simulink model "BuildYourOwnMSD"  (R2024a)
settings: Solver=VariableStepAuto  StartTime=0.0  StopTime=50  MaxStep=0.1  RelTol=1e-3
PreLoadFcn:
  | load Data\MSDParams.mat
undefined symbols (not defined in the file): A, Cd, g, L, m, rho, xdot
libraries: fl_lib x8, nesl_utility x4
CloseFcn:
  | clear
settings Model: Creator=callie  LastModifiedBy=vboutrou
settings DataIOCC: ReturnWorkspaceOutputsName=out3
settings ConfigComp: CovBoundaryAbsTol=1.0e-5

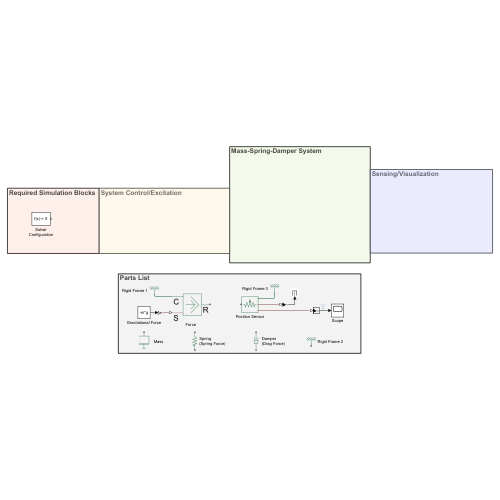
[thumbnail: Simulink's stored preview of the top-level diagram]
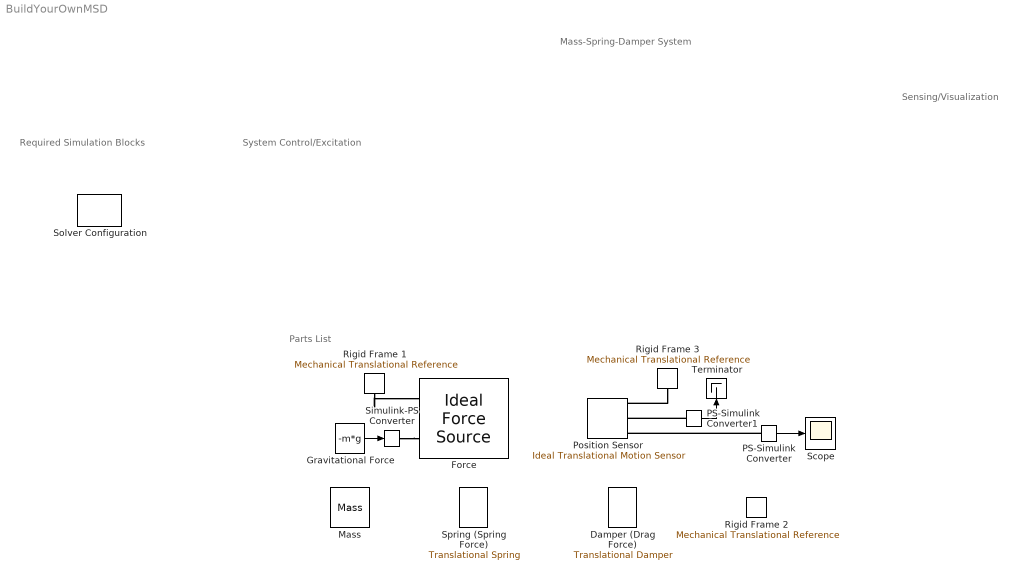
== system BuildYourOwnMSD ==
  note: Required Simulation Blocks
  note: Parts List
  note: Mass-Spring-Damper System
  note: Sensing/Visualization
  note: System Control/Excitation
  Damper (Drag Force) : fl_lib/Mechanical/Translational Elements/Translational Damper  D=0.5*rho*Cd*A*xdot N*s/m  v_specify=off  v_priority=None  v=0 m/s  v_nominal_specify=off  v_nominal_value=1  v_nominal_unit=m/s  f_specify=off  f_priority=None  f=0 N  f_nominal_specify=off  f_nominal_value=1  f_nominal_unit=N
  Force : fl_lib/Mechanical/Mechanical Sources/Ideal Force Source
  Gravitational Force : Constant  Value=-m*g
  Mass : fl_lib/Mechanical/Translational Elements/Mass  mass=m kg  num_ports=foundation.enum.numPorts2.one  v_specify=off  v_priority=High  v=0 m/s  v_nominal_specify=off  v_nominal_value=1  v_nominal_unit=m/s  f_specify=off  f_priority=None  f=0 N  f_nominal_specify=off  f_nominal_value=1  f_nominal_unit=N
  PS-Simulink Converter : nesl_utility/PS-Simulink Converter  PhysicalDomain=network_engine_domain  SubClassName=ps_output  LeftPortType=input  RightPortType=output  PseudoPeriodic=off  Frequencies=[]  VectorFormat=inherit  Unit=m  AffineConversion=off
  PS-Simulink Converter1 : nesl_utility/PS-Simulink Converter  PhysicalDomain=network_engine_domain  SubClassName=ps_output  LeftPortType=input  RightPortType=output  PseudoPeriodic=off  Frequencies=[]  VectorFormat=inherit  Unit=m/s  AffineConversion=off
  Position Sensor : fl_lib/Mechanical/Mechanical Sensors/Ideal Translational Motion Sensor  reference=foundation.enum.MeasurementReference.difference  acceleration_port=false  velocity_port=true  position_port=true  offset=x0 m
  Rigid Frame 1 : fl_lib/Mechanical/Translational Elements/Mechanical Translational Reference
  Rigid Frame 2 : fl_lib/Mechanical/Translational Elements/Mechanical Translational Reference
  Rigid Frame 3 : fl_lib/Mechanical/Translational Elements/Mechanical Translational Reference
  Scope : Scope
  Simulink-PS Converter : nesl_utility/Simulink-PS Converter  PhysicalDomain=network_engine_domain  SubClassName=ps_input  LeftPortType=input  RightPortType=output  PseudoPeriodic=off  Frequencies=[]  NoiseDistribution=none  NoiseParameters=[]  Unit=N  AffineConversion=off  FilteringAndDerivatives=provide  SimscapeFilterOrder=1  InputFilterTimeConstant=0.001  UdotUserProvided=0
  Solver Configuration : nesl_utility/Solver Configuration  PhysicalDomain=network_engine_domain  SubClassName=solver  LeftPortType=input  RightPortType=generic  Tones=[]  Harmonics=[]  SimulateNoise=off  Profile=off  UseLocalSampling=off  EnableSwitchedLinearOptims=on  FrequencyDomain=off  UseCCode=off  RelTol=0.001  AbsTol=0.001  MinStep=1e-09  ToWorkspace=off  RevertToSquareIcSolve=off  NumHomotopyIterations=100  PhasorMode=off  PhasorModeNumHarmonics=1  ConsistencySolver=NEWTON_XTOL_AFTER_FTOL  IndexReductionMethod=DerivativeReplacement  DoDC=off  ResidualTolerance=1e-09  ConsistencyTolSource=GLOBAL  ConsistencyAbsTol=0.001  ConsistencyRelTol=0.001  ConsistencyTolFactor=0.001  UseLocalSolver=off  LocalSolverChoice=NE_BACKWARD_EULER_ADVANCER  ResolveIndetEquations=on  FunctionEvalNumThread=1  LocalSolverSampleTime=0.001  DoFixedCost=off  MaxNonlinIter=3  MaxModeIter=2  ComputeImpulses=off  ImpulseIterations=2  LinearAlgebra=auto  LinearAlgebraNumThread=0  EquationFormulation=NE_TIME_EF  DelaysMemoryBudget=1024  AutomaticFiltering=on  FilteringTimeConstant=0.001  PartitionStorageMethod=AS_NEEDED  PartitionMemoryBudget=1024  PartitionMethod=ROBUST  MultibodyUseLocalSolver=off  MultibodyLocalSolverChoice=ODE1  MultibodyLocalSolverSampleTime=0.001
  Spring (Spring Force) : fl_lib/Mechanical/Translational Elements/Translational Spring  spr_rate=k N/m  v_specify=off  v_priority=None  v=0 m/s  v_nominal_specify=off  v_nominal_value=1  v_nominal_unit=m/s  f_specify=off  f_priority=None  f=0 N  f_nominal_specify=off  f_nominal_value=1  f_nominal_unit=N  x_specify=on  x_priority=High  x=-L m  x_nominal_specify=off  x_nominal_value=1  x_nominal_unit=m
  Terminator : Terminator
  wires:
  PS-Simulink Converter1/1 -> Terminator/1
  PS-Simulink Converter/1 -> Scope/1
  Gravitational Force/1 -> Simulink-PS Converter/1
  connections:
  Simulink-PS Converter/RConn1 -- Force/RConn1
  Rigid Frame 3/LConn1 -- Position Sensor/RConn1
  PS-Simulink Converter/LConn1 -- Position Sensor/RConn3
  PS-Simulink Converter1/LConn1 -- Position Sensor/RConn2
  Rigid Frame 1/LConn1 -- Force/RConn2
